simulink model "PositionControlServoValve"  (R2024b)
settings: Solver=daessc  StartTime=0.0  StopTime=4  MaxStep=0.08  RelTol=1e-3  AbsTol=1e-3
PreLoadFcn:
  | PositionControlServoValveInput
values from neighbouring files (symbols this model uses):
  closePosition = 3e-4    (= 0.0003)    [PositionControlServoValveInput.m]
  dampCoeff = 1e-1    (= 0.1)    [PositionControlServoValveInput.m]
  flapperLength = 5e-3    (= 0.005)    [PositionControlServoValveInput.m]
  flapperRotAngle = 3.4928    [PositionControlServoValveInput.m]
  kii = 0.002    [PositionControlServoValveInput.m]
  kip = 0.004    [PositionControlServoValveInput.m]
  kpi = 600    [PositionControlServoValveInput.m]
  kpp = 160    [PositionControlServoValveInput.m]
  kvi = 10    [PositionControlServoValveInput.m]
  kvp = 200    [PositionControlServoValveInput.m]
  motorC = 1    [PositionControlServoValveInput.m]
  motorDampCoeff = 1e-3    (= 0.001)    [PositionControlServoValveInput.m]
  motorR = 750    [PositionControlServoValveInput.m]
  nozCrossSectArea = (pi/4)*(1.6e-3^2)    (= 2.0106192983e-06)    [PositionControlServoValveInput.m]
  overlap = 0.1    [PositionControlServoValveInput.m]
undefined symbols (not defined in the file or in its folder): smiData, X, Y, Z
libraries: fl_lib x174, sm_lib x50, SimscapeFluids_lib x43, nesl_utility x13
(part 5 of 5)

== system PositionControlServoValve/Position Control Servo Valve/Valve Body1/Orifice BT ==
  Hydraulic Force : fl_lib/Mechanical/Mechanical Sources/Ideal Force Source  Tag=Factory Generic
  MTRef Force : fl_lib/Mechanical/Translational Elements/Mechanical Translational Reference  Tag=Factory Generic
  MTRef Sensor : fl_lib/Mechanical/Translational Elements/Mechanical Translational Reference  Tag=Factory Generic
  Motion Sensor : fl_lib/Mechanical/Mechanical Sensors/Ideal Translational Motion Sensor  Tag=Factory Generic  reference=foundation.enum.MeasurementReference.difference  acceleration_port=false  velocity_port=true  position_port=true  offset=0 m
  Orifice : SimscapeFluids_lib/Isothermal Liquid/Valves & Orifices/Orifices/Spool Orifice (IL)  Tag=Factory Generic  orifice_spec=fluids.isothermal_liquid.valves_orifices.orifices.enum.spool_orifice.rectangle_slot  diameter_hole=5e-3 m  num_hole=6  width=orificeWidth mm  del_S_max="spoolTravel  mm"  S_min=overlap mm  open_orientation=fluids.isothermal_liquid.valves_orifices.enum.spool_orientation.positive  flow_force_spec=simscape.enum.onoff.off  clearance=1e-5 m  area_leak=1e-9 m^2  area=inf m^2  Cd=0.7  Re_c=150  smoothing_factor=0  pressure_recovery=simscape.enum.onoff.off
      settings: InternalSimscapePortConfiguration="{\"Bottom\":[],\"Left\":[{\"id\":\"S\",\"label\":\"S\",\"type\":\"input\"},{\"id\":\"A\",\"label\":\"A\",\"type\":\"foundation.isothermal_liquid.isothermal_liquid\"}],\"Right\":[{\"id\":\"B\",\"label\":\"B\",\"type\":\"foundation.isothermal_liquid.isothermal_liquid\"}],\"Top\":[]}"
  Spool Orifice Hydraulic Force : SimscapeFluids_lib/Isothermal Liquid/Valves & Orifices/Valve Actuators & Forces/Spool Orifice Flow Force (IL)  orifice_spec=fluids.isothermal_liquid.valves_orifices.orifices.enum.spool_orifice.rectangle_slot  diameter_hole=0.005 m  num_hole=4  width=orificeWidth mm  del_S_max="spoolTravel  mm"  S_min=overlap mm  open_orientation=fluids.isothermal_liquid.valves_orifices.enum.spool_orientation.positive  clearance=radClearance mm  area_leak=1e-9 m^2  smoothing_factor=0
      settings: InternalSimscapePortConfiguration="{\"Bottom\":[],\"Left\":[{\"id\":\"A\",\"label\":\"A\",\"type\":\"foundation.isothermal_liquid.isothermal_liquid\"},{\"id\":\"S\",\"label\":\"S\",\"type\":\"input\"}],\"Right\":[{\"id\":\"B\",\"label\":\"B\",\"type\":\"foundation.isothermal_liquid.isothermal_liquid\"},{\"id\":\"F\",\"label\":\"F\",\"type\":\"output\"}],\"Top\":[]}"
  S : PMIOPort  Side=Left
  A : PMIOPort  Port=2  Side=Left
  B : PMIOPort  Port=3  Side=Right
  connections:
  Motion Sensor/RConn3 -- Orifice/LConn1 -- Spool Orifice Hydraulic Force/LConn2
  Hydraulic Force/LConn1 -- Motion Sensor/LConn1 -- S/RConn1
  MTRef Sensor/LConn1 -- Motion Sensor/RConn1
  Orifice/LConn2 -- A/RConn1
  MTRef Force/LConn1 -- Hydraulic Force/RConn2
  Spool Orifice Hydraulic Force/RConn1 -- B/RConn1
  Spool Orifice Hydraulic Force/RConn2 -- Hydraulic Force/RConn1
  Orifice/RConn1 -- Spool Orifice Hydraulic Force/LConn1

== system PositionControlServoValve/Position Control Servo Valve/Valve Body1/Orifice PA ==
  Hydraulic Force : fl_lib/Mechanical/Mechanical Sources/Ideal Force Source  Tag=Factory Generic
  MTRef Force : fl_lib/Mechanical/Translational Elements/Mechanical Translational Reference  Tag=Factory Generic
  MTRef Sensor : fl_lib/Mechanical/Translational Elements/Mechanical Translational Reference  Tag=Factory Generic
  Motion Sensor : fl_lib/Mechanical/Mechanical Sensors/Ideal Translational Motion Sensor  Tag=Factory Generic  reference=foundation.enum.MeasurementReference.difference  acceleration_port=false  velocity_port=true  position_port=true  offset=0 m
  Orifice : SimscapeFluids_lib/Isothermal Liquid/Valves & Orifices/Orifices/Spool Orifice (IL)  Tag=Factory Generic  orifice_spec=fluids.isothermal_liquid.valves_orifices.orifices.enum.spool_orifice.rectangle_slot  diameter_hole=5e-3 m  num_hole=6  width=orificeWidth mm  del_S_max="spoolTravel  mm"  S_min=overlap mm  open_orientation=fluids.isothermal_liquid.valves_orifices.enum.spool_orientation.positive  flow_force_spec=simscape.enum.onoff.off  clearance=1e-5 m  area_leak=1e-9 m^2  area=inf m^2  Cd=0.7  Re_c=150  smoothing_factor=0  pressure_recovery=simscape.enum.onoff.off
      settings: InternalSimscapePortConfiguration="{\"Bottom\":[],\"Left\":[{\"id\":\"S\",\"label\":\"S\",\"type\":\"input\"},{\"id\":\"A\",\"label\":\"A\",\"type\":\"foundation.isothermal_liquid.isothermal_liquid\"}],\"Right\":[{\"id\":\"B\",\"label\":\"B\",\"type\":\"foundation.isothermal_liquid.isothermal_liquid\"}],\"Top\":[]}"
  Spool Orifice Hydraulic Force : SimscapeFluids_lib/Isothermal Liquid/Valves & Orifices/Valve Actuators & Forces/Spool Orifice Flow Force (IL)  orifice_spec=fluids.isothermal_liquid.valves_orifices.orifices.enum.spool_orifice.rectangle_slot  diameter_hole=0.005 m  num_hole=4  width=orificeWidth mm  del_S_max="spoolTravel  mm"  S_min=overlap mm  open_orientation=fluids.isothermal_liquid.valves_orifices.enum.spool_orientation.positive  clearance=radClearance mm  area_leak=1e-9 m^2  smoothing_factor=0
      settings: InternalSimscapePortConfiguration="{\"Bottom\":[],\"Left\":[{\"id\":\"A\",\"label\":\"A\",\"type\":\"foundation.isothermal_liquid.isothermal_liquid\"},{\"id\":\"S\",\"label\":\"S\",\"type\":\"input\"}],\"Right\":[{\"id\":\"B\",\"label\":\"B\",\"type\":\"foundation.isothermal_liquid.isothermal_liquid\"},{\"id\":\"F\",\"label\":\"F\",\"type\":\"output\"}],\"Top\":[]}"
  S : PMIOPort  Side=Left
  A : PMIOPort  Port=2  Side=Left
  B : PMIOPort  Port=3  Side=Right
  connections:
  Spool Orifice Hydraulic Force/RConn2 -- Hydraulic Force/RConn1
  Spool Orifice Hydraulic Force/LConn1 -- Orifice/RConn1
  A/RConn1 -- Orifice/LConn2
  Spool Orifice Hydraulic Force/RConn1 -- B/RConn1
  Spool Orifice Hydraulic Force/LConn2 -- Motion Sensor/RConn3 -- Orifice/LConn1
  MTRef Sensor/LConn1 -- Motion Sensor/RConn1
  MTRef Force/LConn1 -- Hydraulic Force/RConn2
  S/RConn1 -- Motion Sensor/LConn1 -- Hydraulic Force/LConn1

== system PositionControlServoValve/Position Control Servo Valve/Valve Body1/Orifice PB ==
  Hydraulic Force : fl_lib/Mechanical/Mechanical Sources/Ideal Force Source  Tag=Factory Generic
  MTRef Force : fl_lib/Mechanical/Translational Elements/Mechanical Translational Reference  Tag=Factory Generic
  MTRef Sensor : fl_lib/Mechanical/Translational Elements/Mechanical Translational Reference  Tag=Factory Generic
  Motion Sensor : fl_lib/Mechanical/Mechanical Sensors/Ideal Translational Motion Sensor  Tag=Factory Generic  reference=foundation.enum.MeasurementReference.difference  acceleration_port=false  velocity_port=true  position_port=true  offset=0 m
  Orifice : SimscapeFluids_lib/Isothermal Liquid/Valves & Orifices/Orifices/Spool Orifice (IL)  Tag=Factory Generic  orifice_spec=fluids.isothermal_liquid.valves_orifices.orifices.enum.spool_orifice.rectangle_slot  diameter_hole=5e-3 m  num_hole=6  width=orificeWidth mm  del_S_max="spoolTravel  mm"  S_min=-overlap mm  open_orientation=fluids.isothermal_liquid.valves_orifices.enum.spool_orientation.negative  flow_force_spec=simscape.enum.onoff.off  clearance=1e-5 m  area_leak=1e-9 m^2  area=inf m^2  Cd=0.7  Re_c=150  smoothing_factor=0  pressure_recovery=simscape.enum.onoff.off
      settings: InternalSimscapePortConfiguration="{\"Bottom\":[],\"Left\":[{\"id\":\"S\",\"label\":\"S\",\"type\":\"input\"},{\"id\":\"A\",\"label\":\"A\",\"type\":\"foundation.isothermal_liquid.isothermal_liquid\"}],\"Right\":[{\"id\":\"B\",\"label\":\"B\",\"type\":\"foundation.isothermal_liquid.isothermal_liquid\"}],\"Top\":[]}"
  Spool Orifice Hydraulic Force : SimscapeFluids_lib/Isothermal Liquid/Valves & Orifices/Valve Actuators & Forces/Spool Orifice Flow Force (IL)  orifice_spec=fluids.isothermal_liquid.valves_orifices.orifices.enum.spool_orifice.rectangle_slot  diameter_hole=0.005 m  num_hole=4  width=orificeWidth mm  del_S_max="spoolTravel  mm"  S_min=-overlap mm  open_orientation=fluids.isothermal_liquid.valves_orifices.enum.spool_orientation.negative  clearance=radClearance mm  area_leak=1e-9 m^2  smoothing_factor=0
      settings: InternalSimscapePortConfiguration="{\"Bottom\":[],\"Left\":[{\"id\":\"A\",\"label\":\"A\",\"type\":\"foundation.isothermal_liquid.isothermal_liquid\"},{\"id\":\"S\",\"label\":\"S\",\"type\":\"input\"}],\"Right\":[{\"id\":\"B\",\"label\":\"B\",\"type\":\"foundation.isothermal_liquid.isothermal_liquid\"},{\"id\":\"F\",\"label\":\"F\",\"type\":\"output\"}],\"Top\":[]}"
  S : PMIOPort  Side=Left
  A : PMIOPort  Port=2  Side=Left
  B : PMIOPort  Port=3  Side=Right
  connections:
  Motion Sensor/RConn3 -- Orifice/LConn1 -- Spool Orifice Hydraulic Force/LConn2
  S/RConn1 -- Motion Sensor/LConn1 -- Hydraulic Force/LConn1
  Spool Orifice Hydraulic Force/RConn2 -- Hydraulic Force/RConn1
  Orifice/LConn2 -- A/RConn1
  MTRef Force/LConn1 -- Hydraulic Force/RConn2
  MTRef Sensor/LConn1 -- Motion Sensor/RConn1
  Orifice/RConn1 -- Spool Orifice Hydraulic Force/LConn1
  Spool Orifice Hydraulic Force/RConn1 -- B/RConn1

== system PositionControlServoValve/Position Control Servo Valve/Valve Body2/Orifice AT ==
  Hydraulic Force : fl_lib/Mechanical/Mechanical Sources/Ideal Force Source  Tag=Factory Generic
  MTRef Force : fl_lib/Mechanical/Translational Elements/Mechanical Translational Reference  Tag=Factory Generic
  MTRef Sensor : fl_lib/Mechanical/Translational Elements/Mechanical Translational Reference  Tag=Factory Generic
  Motion Sensor : fl_lib/Mechanical/Mechanical Sensors/Ideal Translational Motion Sensor  Tag=Factory Generic  reference=foundation.enum.MeasurementReference.difference  acceleration_port=false  velocity_port=true  position_port=true  offset=0 m
  Orifice : SimscapeFluids_lib/Isothermal Liquid/Valves & Orifices/Orifices/Spool Orifice (IL)  Tag=Factory Generic  orifice_spec=fluids.isothermal_liquid.valves_orifices.orifices.enum.spool_orifice.rectangle_slot  diameter_hole=5e-3 m  num_hole=6  width=orificeWidth mm  del_S_max="spoolTravel  mm"  S_min=-overlap mm  open_orientation=fluids.isothermal_liquid.valves_orifices.enum.spool_orientation.negative  flow_force_spec=simscape.enum.onoff.off  clearance=1e-5 m  area_leak=1e-9 m^2  area=inf m^2  Cd=0.7  Re_c=150  smoothing_factor=0  pressure_recovery=simscape.enum.onoff.off
      settings: InternalSimscapePortConfiguration="{\"Bottom\":[],\"Left\":[{\"id\":\"S\",\"label\":\"S\",\"type\":\"input\"},{\"id\":\"A\",\"label\":\"A\",\"type\":\"foundation.isothermal_liquid.isothermal_liquid\"}],\"Right\":[{\"id\":\"B\",\"label\":\"B\",\"type\":\"foundation.isothermal_liquid.isothermal_liquid\"}],\"Top\":[]}"
  Spool Orifice Hydraulic Force : SimscapeFluids_lib/Isothermal Liquid/Valves & Orifices/Valve Actuators & Forces/Spool Orifice Flow Force (IL)  orifice_spec=fluids.isothermal_liquid.valves_orifices.orifices.enum.spool_orifice.rectangle_slot  diameter_hole=0.005 m  num_hole=4  width=orificeWidth mm  del_S_max="spoolTravel  mm"  S_min=-overlap mm  open_orientation=fluids.isothermal_liquid.valves_orifices.enum.spool_orientation.negative  clearance=radClearance mm  area_leak=1e-9 m^2  smoothing_factor=0
      settings: InternalSimscapePortConfiguration="{\"Bottom\":[],\"Left\":[{\"id\":\"A\",\"label\":\"A\",\"type\":\"foundation.isothermal_liquid.isothermal_liquid\"},{\"id\":\"S\",\"label\":\"S\",\"type\":\"input\"}],\"Right\":[{\"id\":\"B\",\"label\":\"B\",\"type\":\"foundation.isothermal_liquid.isothermal_liquid\"},{\"id\":\"F\",\"label\":\"F\",\"type\":\"output\"}],\"Top\":[]}"
  S : PMIOPort  Side=Left
  A : PMIOPort  Port=2  Side=Left
  B : PMIOPort  Port=3  Side=Right
  connections:
  Motion Sensor/RConn3 -- Orifice/LConn1 -- Spool Orifice Hydraulic Force/LConn2
  Hydraulic Force/LConn1 -- Motion Sensor/LConn1 -- S/RConn1
  Orifice/RConn1 -- Spool Orifice Hydraulic Force/LConn1
  Orifice/LConn2 -- A/RConn1
  MTRef Force/LConn1 -- Hydraulic Force/RConn2
  MTRef Sensor/LConn1 -- Motion Sensor/RConn1
  Spool Orifice Hydraulic Force/RConn2 -- Hydraulic Force/RConn1
  Spool Orifice Hydraulic Force/RConn1 -- B/RConn1

== system PositionControlServoValve/Position Control Servo Valve/Valve Body2/Orifice BT ==
  Hydraulic Force : fl_lib/Mechanical/Mechanical Sources/Ideal Force Source  Tag=Factory Generic
  MTRef Force : fl_lib/Mechanical/Translational Elements/Mechanical Translational Reference  Tag=Factory Generic
  MTRef Sensor : fl_lib/Mechanical/Translational Elements/Mechanical Translational Reference  Tag=Factory Generic
  Motion Sensor : fl_lib/Mechanical/Mechanical Sensors/Ideal Translational Motion Sensor  Tag=Factory Generic  reference=foundation.enum.MeasurementReference.difference  acceleration_port=false  velocity_port=true  position_port=true  offset=0 m
  Orifice : SimscapeFluids_lib/Isothermal Liquid/Valves & Orifices/Orifices/Spool Orifice (IL)  Tag=Factory Generic  orifice_spec=fluids.isothermal_liquid.valves_orifices.orifices.enum.spool_orifice.rectangle_slot  diameter_hole=5e-3 m  num_hole=6  width=orificeWidth mm  del_S_max="spoolTravel  mm"  S_min=overlap mm  open_orientation=fluids.isothermal_liquid.valves_orifices.enum.spool_orientation.positive  flow_force_spec=simscape.enum.onoff.off  clearance=1e-5 m  area_leak=1e-9 m^2  area=inf m^2  Cd=0.7  Re_c=150  smoothing_factor=0  pressure_recovery=simscape.enum.onoff.off
      settings: InternalSimscapePortConfiguration="{\"Bottom\":[],\"Left\":[{\"id\":\"S\",\"label\":\"S\",\"type\":\"input\"},{\"id\":\"A\",\"label\":\"A\",\"type\":\"foundation.isothermal_liquid.isothermal_liquid\"}],\"Right\":[{\"id\":\"B\",\"label\":\"B\",\"type\":\"foundation.isothermal_liquid.isothermal_liquid\"}],\"Top\":[]}"
  Spool Orifice Hydraulic Force : SimscapeFluids_lib/Isothermal Liquid/Valves & Orifices/Valve Actuators & Forces/Spool Orifice Flow Force (IL)  orifice_spec=fluids.isothermal_liquid.valves_orifices.orifices.enum.spool_orifice.rectangle_slot  diameter_hole=0.005 m  num_hole=4  width=orificeWidth mm  del_S_max="spoolTravel  mm"  S_min=overlap mm  open_orientation=fluids.isothermal_liquid.valves_orifices.enum.spool_orientation.positive  clearance=radClearance mm  area_leak=1e-9 m^2  smoothing_factor=0
      settings: InternalSimscapePortConfiguration="{\"Bottom\":[],\"Left\":[{\"id\":\"A\",\"label\":\"A\",\"type\":\"foundation.isothermal_liquid.isothermal_liquid\"},{\"id\":\"S\",\"label\":\"S\",\"type\":\"input\"}],\"Right\":[{\"id\":\"B\",\"label\":\"B\",\"type\":\"foundation.isothermal_liquid.isothermal_liquid\"},{\"id\":\"F\",\"label\":\"F\",\"type\":\"output\"}],\"Top\":[]}"
  S : PMIOPort  Side=Left
  A : PMIOPort  Port=2  Side=Left
  B : PMIOPort  Port=3  Side=Right
  connections:
  Motion Sensor/RConn3 -- Orifice/LConn1 -- Spool Orifice Hydraulic Force/LConn2
  Hydraulic Force/LConn1 -- Motion Sensor/LConn1 -- S/RConn1
  MTRef Sensor/LConn1 -- Motion Sensor/RConn1
  Orifice/LConn2 -- A/RConn1
  MTRef Force/LConn1 -- Hydraulic Force/RConn2
  Spool Orifice Hydraulic Force/RConn1 -- B/RConn1
  Spool Orifice Hydraulic Force/RConn2 -- Hydraulic Force/RConn1
  Orifice/RConn1 -- Spool Orifice Hydraulic Force/LConn1

== system PositionControlServoValve/Position Control Servo Valve/Valve Body2/Orifice PA ==
  Hydraulic Force : fl_lib/Mechanical/Mechanical Sources/Ideal Force Source  Tag=Factory Generic
  MTRef Force : fl_lib/Mechanical/Translational Elements/Mechanical Translational Reference  Tag=Factory Generic
  MTRef Sensor : fl_lib/Mechanical/Translational Elements/Mechanical Translational Reference  Tag=Factory Generic
  Motion Sensor : fl_lib/Mechanical/Mechanical Sensors/Ideal Translational Motion Sensor  Tag=Factory Generic  reference=foundation.enum.MeasurementReference.difference  acceleration_port=false  velocity_port=true  position_port=true  offset=0 m
  Orifice : SimscapeFluids_lib/Isothermal Liquid/Valves & Orifices/Orifices/Spool Orifice (IL)  Tag=Factory Generic  orifice_spec=fluids.isothermal_liquid.valves_orifices.orifices.enum.spool_orifice.rectangle_slot  diameter_hole=5e-3 m  num_hole=6  width=orificeWidth mm  del_S_max="spoolTravel  mm"  S_min=overlap mm  open_orientation=fluids.isothermal_liquid.valves_orifices.enum.spool_orientation.positive  flow_force_spec=simscape.enum.onoff.off  clearance=1e-5 m  area_leak=1e-9 m^2  area=inf m^2  Cd=0.7  Re_c=150  smoothing_factor=0  pressure_recovery=simscape.enum.onoff.off
      settings: InternalSimscapePortConfiguration="{\"Bottom\":[],\"Left\":[{\"id\":\"S\",\"label\":\"S\",\"type\":\"input\"},{\"id\":\"A\",\"label\":\"A\",\"type\":\"foundation.isothermal_liquid.isothermal_liquid\"}],\"Right\":[{\"id\":\"B\",\"label\":\"B\",\"type\":\"foundation.isothermal_liquid.isothermal_liquid\"}],\"Top\":[]}"
  Spool Orifice Hydraulic Force : SimscapeFluids_lib/Isothermal Liquid/Valves & Orifices/Valve Actuators & Forces/Spool Orifice Flow Force (IL)  orifice_spec=fluids.isothermal_liquid.valves_orifices.orifices.enum.spool_orifice.rectangle_slot  diameter_hole=0.005 m  num_hole=4  width=orificeWidth mm  del_S_max="spoolTravel  mm"  S_min=overlap mm  open_orientation=fluids.isothermal_liquid.valves_orifices.enum.spool_orientation.positive  clearance=radClearance mm  area_leak=1e-9 m^2  smoothing_factor=0
      settings: InternalSimscapePortConfiguration="{\"Bottom\":[],\"Left\":[{\"id\":\"A\",\"label\":\"A\",\"type\":\"foundation.isothermal_liquid.isothermal_liquid\"},{\"id\":\"S\",\"label\":\"S\",\"type\":\"input\"}],\"Right\":[{\"id\":\"B\",\"label\":\"B\",\"type\":\"foundation.isothermal_liquid.isothermal_liquid\"},{\"id\":\"F\",\"label\":\"F\",\"type\":\"output\"}],\"Top\":[]}"
  S : PMIOPort  Side=Left
  A : PMIOPort  Port=2  Side=Left
  B : PMIOPort  Port=3  Side=Right
  connections:
  Spool Orifice Hydraulic Force/RConn2 -- Hydraulic Force/RConn1
  Spool Orifice Hydraulic Force/LConn1 -- Orifice/RConn1
  A/RConn1 -- Orifice/LConn2
  Spool Orifice Hydraulic Force/RConn1 -- B/RConn1
  Spool Orifice Hydraulic Force/LConn2 -- Motion Sensor/RConn3 -- Orifice/LConn1
  MTRef Sensor/LConn1 -- Motion Sensor/RConn1
  MTRef Force/LConn1 -- Hydraulic Force/RConn2
  S/RConn1 -- Motion Sensor/LConn1 -- Hydraulic Force/LConn1

== system PositionControlServoValve/Position Control Servo Valve/Valve Body2/Orifice PB ==
  Hydraulic Force : fl_lib/Mechanical/Mechanical Sources/Ideal Force Source  Tag=Factory Generic
  MTRef Force : fl_lib/Mechanical/Translational Elements/Mechanical Translational Reference  Tag=Factory Generic
  MTRef Sensor : fl_lib/Mechanical/Translational Elements/Mechanical Translational Reference  Tag=Factory Generic
  Motion Sensor : fl_lib/Mechanical/Mechanical Sensors/Ideal Translational Motion Sensor  Tag=Factory Generic  reference=foundation.enum.MeasurementReference.difference  acceleration_port=false  velocity_port=true  position_port=true  offset=0 m
  Orifice : SimscapeFluids_lib/Isothermal Liquid/Valves & Orifices/Orifices/Spool Orifice (IL)  Tag=Factory Generic  orifice_spec=fluids.isothermal_liquid.valves_orifices.orifices.enum.spool_orifice.rectangle_slot  diameter_hole=5e-3 m  num_hole=6  width=orificeWidth mm  del_S_max="spoolTravel  mm"  S_min=-overlap mm  open_orientation=fluids.isothermal_liquid.valves_orifices.enum.spool_orientation.negative  flow_force_spec=simscape.enum.onoff.off  clearance=1e-5 m  area_leak=1e-9 m^2  area=inf m^2  Cd=0.7  Re_c=150  smoothing_factor=0  pressure_recovery=simscape.enum.onoff.off
      settings: InternalSimscapePortConfiguration="{\"Bottom\":[],\"Left\":[{\"id\":\"S\",\"label\":\"S\",\"type\":\"input\"},{\"id\":\"A\",\"label\":\"A\",\"type\":\"foundation.isothermal_liquid.isothermal_liquid\"}],\"Right\":[{\"id\":\"B\",\"label\":\"B\",\"type\":\"foundation.isothermal_liquid.isothermal_liquid\"}],\"Top\":[]}"
  Spool Orifice Hydraulic Force : SimscapeFluids_lib/Isothermal Liquid/Valves & Orifices/Valve Actuators & Forces/Spool Orifice Flow Force (IL)  orifice_spec=fluids.isothermal_liquid.valves_orifices.orifices.enum.spool_orifice.rectangle_slot  diameter_hole=0.005 m  num_hole=4  width=orificeWidth mm  del_S_max="spoolTravel  mm"  S_min=-overlap mm  open_orientation=fluids.isothermal_liquid.valves_orifices.enum.spool_orientation.negative  clearance=radClearance mm  area_leak=1e-9 m^2  smoothing_factor=0
      settings: InternalSimscapePortConfiguration="{\"Bottom\":[],\"Left\":[{\"id\":\"A\",\"label\":\"A\",\"type\":\"foundation.isothermal_liquid.isothermal_liquid\"},{\"id\":\"S\",\"label\":\"S\",\"type\":\"input\"}],\"Right\":[{\"id\":\"B\",\"label\":\"B\",\"type\":\"foundation.isothermal_liquid.isothermal_liquid\"},{\"id\":\"F\",\"label\":\"F\",\"type\":\"output\"}],\"Top\":[]}"
  S : PMIOPort  Side=Left
  A : PMIOPort  Port=2  Side=Left
  B : PMIOPort  Port=3  Side=Right
  connections:
  Motion Sensor/RConn3 -- Orifice/LConn1 -- Spool Orifice Hydraulic Force/LConn2
  S/RConn1 -- Motion Sensor/LConn1 -- Hydraulic Force/LConn1
  Spool Orifice Hydraulic Force/RConn2 -- Hydraulic Force/RConn1
  Orifice/LConn2 -- A/RConn1
  MTRef Force/LConn1 -- Hydraulic Force/RConn2
  MTRef Sensor/LConn1 -- Motion Sensor/RConn1
  Orifice/RConn1 -- Spool Orifice Hydraulic Force/LConn1
  Spool Orifice Hydraulic Force/RConn1 -- B/RConn1
